simulink model "classic_sound_tuner"  (R2026a)
settings: Solver=FixedStepDiscrete  StopTime=5  FixedStep=0.01
InitFcn:
  | run('E:\Tesla_speed\prj\tools\sound_sim\simulink\init_sound_tuner_model.m')
values from neighbouring files (symbols this model uses):
  GearCmd = 2    [init_sound_tuner_model.m]
  OverallRatio = GearRatios(GearCmd) * FinalDrive    [init_sound_tuner_model.m]
  RedlineRPM = profile.redline_rpm    [init_sound_tuner_model.m]
  ShiftGainCmd = 1.0    (= 1)    [init_sound_tuner_model.m]
  SpeedKmh = 80    [init_sound_tuner_model.m]
  ThrottleCmd = 0.65    [init_sound_tuner_model.m]
  WheelRadiusM = profile.wheel_radius_m    [init_sound_tuner_model.m]
settings Model: Creator=Jovi  LastModifiedBy=Jovi

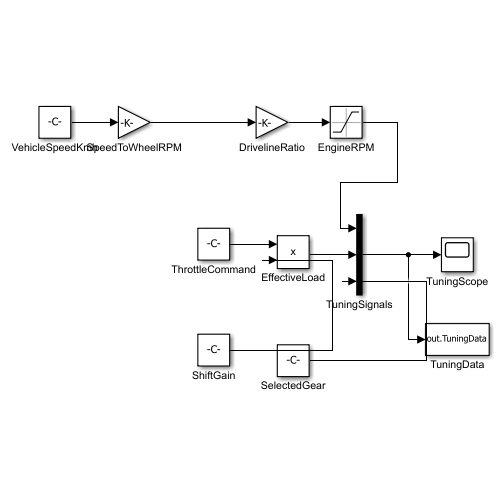
[thumbnail: Simulink's stored preview of the top-level diagram]
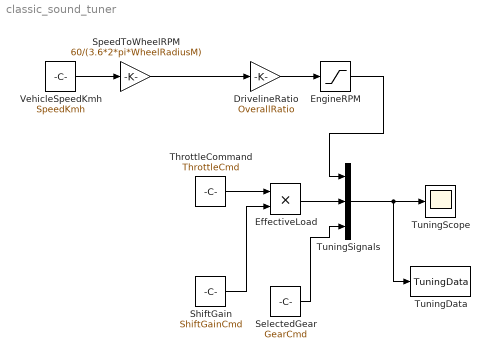
== system classic_sound_tuner ==
  DrivelineRatio : Gain  Gain=OverallRatio
  EffectiveLoad : Product
  EngineRPM : Saturate  UpperLimit=RedlineRPM  LowerLimit=0
  SelectedGear : Constant  Value=GearCmd
  ShiftGain : Constant  Value=ShiftGainCmd
  SpeedToWheelRPM : Gain  Gain=60/(3.6*2*pi*WheelRadiusM)
  ThrottleCommand : Constant  Value=ThrottleCmd
  TuningData : ToWorkspace  VariableName=TuningData  SaveFormat=Structure With Time  SampleTime=-1
  TuningScope : Scope
  TuningSignals : Mux  Inputs=3
  VehicleSpeedKmh : Constant  Value=SpeedKmh
  wires:
  TuningSignals/1 -> TuningData/1, TuningScope/1
  SelectedGear/1 -> TuningSignals/3
  EffectiveLoad/1 -> TuningSignals/2
  EngineRPM/1 -> TuningSignals/1
  ShiftGain/1 -> EffectiveLoad/2
  ThrottleCommand/1 -> EffectiveLoad/1
  DrivelineRatio/1 -> EngineRPM/1
  SpeedToWheelRPM/1 -> DrivelineRatio/1
  VehicleSpeedKmh/1 -> SpeedToWheelRPM/1
